simulink model "ur_servo"  (R2022b)
settings: Solver=FixedStepAuto  StartTime=0.0  StopTime=inf  RelTol=1e-3
model workspace (MAT data in the model file):
  SL_ROS_VariableLengthArrays_MaxSizes.CommonInfo.ArrayTruncateAction = 'EmitWarning'
  SL_ROS_VariableLengthArrays_MaxSizes.MsgTypeMap = containers.Map
  SL_ROS_VariableLengthArrays_MaxSizes.MsgTypeMap.serialization.keys = {'sensor_msgs/Image', 'std_msgs/Float64MultiArray', 'tf2_msgs/TFMessage'}
  SL_ROS_VariableLengthArrays_MaxSizes.MsgTypeMap.serialization.values{1}(1).PropertyName = 'Data'
  SL_ROS_VariableLengthArrays_MaxSizes.MsgTypeMap.serialization.values{1}(1).DataType = 'uint8'
  SL_ROS_VariableLengthArrays_MaxSizes.MsgTypeMap.serialization.values{1}(1).MaxLength = 921600
  SL_ROS_VariableLengthArrays_MaxSizes.MsgTypeMap.serialization.values{1}(2).PropertyName = 'Encoding'
  SL_ROS_VariableLengthArrays_MaxSizes.MsgTypeMap.serialization.values{1}(2).DataType = 'uint8'
  SL_ROS_VariableLengthArrays_MaxSizes.MsgTypeMap.serialization.values{1}(2).MaxLength = 921600
  SL_ROS_VariableLengthArrays_MaxSizes.MsgTypeMap.serialization.values{2}.PropertyName = 'Data'
  SL_ROS_VariableLengthArrays_MaxSizes.MsgTypeMap.serialization.values{2}.DataType = 'double'
  SL_ROS_VariableLengthArrays_MaxSizes.MsgTypeMap.serialization.values{2}.MaxLength = 16
  SL_ROS_VariableLengthArrays_MaxSizes.MsgTypeMap.serialization.values{3}.PropertyName = 'Transforms'
  SL_ROS_VariableLengthArrays_MaxSizes.MsgTypeMap.serialization.values{3}.DataType = 'geometry_msgs/TransformStamped'
  SL_ROS_VariableLengthArrays_MaxSizes.MsgTypeMap.serialization.values{3}.MaxLength = 1
  SL_ROS_VariableLengthArrays_MaxSizes.MsgTypeMap.serialization.uniformity = 0
  SL_ROS_VariableLengthArrays_MaxSizes.MsgTypeMap.serialization.keyType = 'char'
  SL_ROS_VariableLengthArrays_MaxSizes.MsgTypeMap.serialization.valueType = 'any'
undefined symbols (not defined in the file or in its folder): Angular, Linear
libraries: robotlib x10
settings Model: Creator=user  LastModifiedBy=16122
settings OptimizationCC: EnhancedBackFolding=on  PassReuseOutputArgsAs=Individual arguments  ZeroExternalMemoryAtStartup=off  ZeroInternalMemoryAtStartup=off  MaxStackSize=64  OptimizeBlockOrder=speed  DifferentSizesBufferReuse=on  OptimizationCustomize=off  EfficientTunableParamExpr=on
settings DebuggingCC: ParameterTunabilityLossMsg=error
settings HardwareCC: ProdBitPerPointer=32  ProdBitPerSizeT=32  ProdBitPerPtrDiffT=32  ProdLargestAtomicFloat=None  ProdIntDivRoundTo=Undefined  ProdEndianess=Unspecified  ProdWordSize=32  ProdHWDeviceType=Generic->Unspecified (assume 32-bit Generic)
settings SFSimCC: MATLABDynamicMemAlloc=off
settings RTWCC: Description=Embedded Coder  SystemTargetFile=ert.tlc  HardwareBoard=Robot Operating System (ROS)  TLCOptions="-aInlineSetEventsForThisBaseRateFcn=TLC_FALSE -aSuppressMultiTaskScheduler=TLC_FALSE  -aRateBasedStepFcn=0"  TemplateMakefile=ert_default_tmf  Toolchain=Catkin  TargetLang=C++
settings CodeAppCC: ForceParamTrailComments=on  IgnoreCustomStorageClasses=off  OperatorAnnotations=on  SimulinkDataObjDesc=on  SFDataObjDesc=on  InsertBlockDesc=on

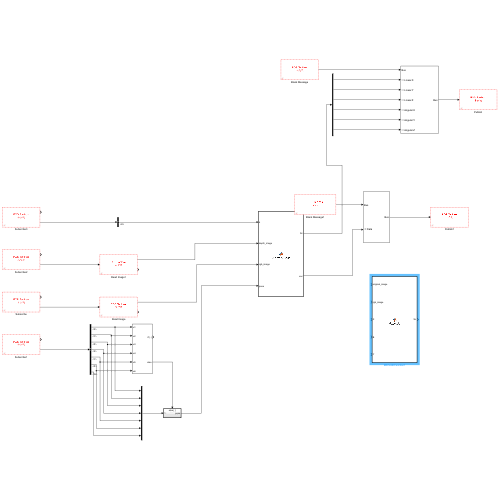
[thumbnail: Simulink's stored preview of the top-level diagram]
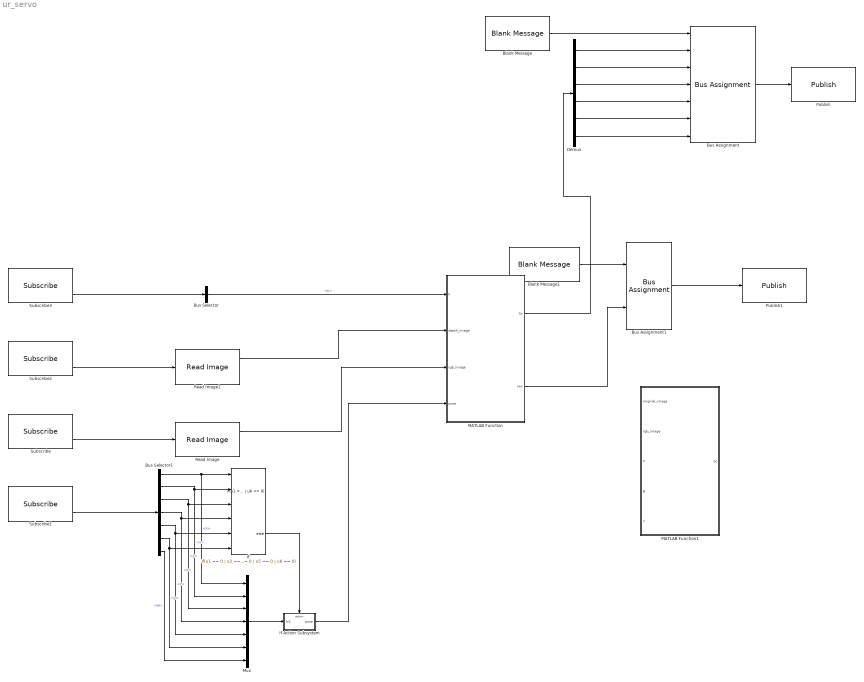
== system ur_servo ==
  Blank Message : robotlib/Blank Message  messageClass=Message  entityType=geometry_msgs/Twist  messageType=geometry_msgs/Twist  SampleTime=inf  legacyBusStruct=off
      settings: LibrarySourceBlock=roslib/ROS/Blank Message
  Blank Message1 : robotlib/Blank Message  messageClass=Message  entityType=std_msgs/Float64MultiArray  messageType=std_msgs/Float64MultiArray  SampleTime=inf  legacyBusStruct=off
      settings: LibrarySourceBlock=roslib/ROS/Blank Message
  Bus Assignment : BusAssignment  AssignedSignals=Linear.X,Linear.Y,Linear.Z,Angular.X,Angular.Y,Angular.Z
  Bus Assignment1 : BusAssignment  AssignedSignals=Data
  Bus Selector : BusSelector  OutputSignals=K
  Bus Selector1 : BusSelector  OutputSignals=Transforms.Transform.Translation.X,Transforms.Transform.Translation.Y,Transforms.Transform.Translation.Z,Transforms.Transform.Rotation.X,Transforms.Transform.Rotation.Y,Transforms.Transform.Rotation.Z,Transforms.Transform.Rotation.W
  Demux : Demux  Outputs=6
  If : If  NumInputs=6  IfExpression=u1 == 0 | u2 == 0 | u3 == 0 | u4 == 0 | u5 == 0 | u6 == 0
  If Action Subsystem : Subsystem  TreatAsAtomicUnit=on
  MATLAB Function : MATLAB Function  TreatAsAtomicUnit=on
  MATLAB Function1 : MATLAB Function  TreatAsAtomicUnit=on
  Mux : Mux  Inputs=7
  Publish : robotlib/Publish  topicSource=Select from ROS network  topic=/twist_controller/command  messageType=geometry_msgs/Twist  legacyBusStruct=off  messageQueueLength=1
      settings: LibrarySourceBlock=roslib/ROS/Publish
  Publish1 : robotlib/Publish  topicSource=Specify your own  topic=/urx  messageType=std_msgs/Float64MultiArray  legacyBusStruct=off  messageQueueLength=1
      settings: LibrarySourceBlock=roslib/ROS/Publish
  Read Image : robotlib/Read Image  MaximumImageSize=[480, 640]  ImageEncoding=rgb8  ShowAlphaOutput=off  ShowErrorCodeOutput=on  VariableSizeOutputs=off
      settings: LibrarySourceBlock=roslib/ROS/Read Image
  Read Image1 : robotlib/Read Image  MaximumImageSize=[480, 640]  ImageEncoding=16uc1  ShowAlphaOutput=off  ShowErrorCodeOutput=on  VariableSizeOutputs=off
      settings: LibrarySourceBlock=roslib/ROS/Read Image
  Subscribe : robotlib/Subscribe  topicSource=Select from ROS network  topic=/camera/color/image_raw  messageType=sensor_msgs/Image  SampleTime=-1  legacyBusStruct=off  messageQueueLength=1
      settings: LibrarySourceBlock=roslib/ROS/Subscribe
  Subscribe1 : robotlib/Subscribe  topicSource=Select from ROS network  topic=/tf  messageType=tf2_msgs/TFMessage  SampleTime=-1  legacyBusStruct=off  messageQueueLength=1
      settings: LibrarySourceBlock=roslib/ROS/Subscribe
  Subscribe2 : robotlib/Subscribe  topicSource=Select from ROS network  topic=/camera/aligned_depth_to_color/image_raw  messageType=sensor_msgs/Image  SampleTime=-1  legacyBusStruct=off  messageQueueLength=1
      settings: LibrarySourceBlock=roslib/ROS/Subscribe
  Subscribe3 : robotlib/Subscribe  topicSource=Select from ROS network  topic=/camera/color/camera_info  messageType=sensor_msgs/CameraInfo  SampleTime=-1  legacyBusStruct=off  messageQueueLength=1
      settings: LibrarySourceBlock=roslib/ROS/Subscribe
  wires:
  Subscribe/2 -> Read Image/1
  Read Image/1 -> MATLAB Function/3(rgb_image)
  Bus Selector1/1 -> Mux/1, If/1  "<X>"
  Bus Selector1/2 -> If/2, Mux/2  "<Y>"
  Bus Selector1/3 -> If/3, Mux/3  "<Z>"
  Bus Selector1/4 -> Mux/4, If/4  "<X>"
  Bus Selector1/5 -> Mux/5, If/5  "<Y>"
  Bus Selector1/6 -> If/6, Mux/6  "<Z>"
  If/2 -> If Action Subsystem/Action
  Subscribe2/2 -> Read Image1/1
  Read Image1/1 -> MATLAB Function/2(depth_image)
  Subscribe1/2 -> Bus Selector1/1
  Mux/1 -> If Action Subsystem/1(In1)
  If Action Subsystem/1(pose) -> MATLAB Function/4(pose)
  Subscribe3/2 -> Bus Selector/1
  Bus Selector/1 -> MATLAB Function/1(k)  "<K>"
  Blank Message/1 -> Bus Assignment/1
  Bus Assignment/1 -> Publish/1
  MATLAB Function/1(Sc) -> Demux/1
  Demux/1 -> Bus Assignment/2
  Demux/2 -> Bus Assignment/3
  Demux/3 -> Bus Assignment/4
  Demux/4 -> Bus Assignment/5
  Demux/5 -> Bus Assignment/6
  Demux/6 -> Bus Assignment/7
  Bus Selector1/7 -> Mux/7  "<W>"
  Blank Message1/1 -> Bus Assignment1/1
  MATLAB Function/2(vec) -> Bus Assignment1/2
  Bus Assignment1/1 -> Publish1/1

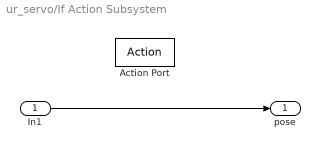
== system ur_servo/If Action Subsystem ==
  In1 : Inport
  Action Port : ActionPort  ActionPortLabel=else
  pose : Outport
  wires:
  In1/1 -> pose/1

== matlab function ur_servo/MATLAB Function1 ==
  data: original_image input; rgb_image input; Sc output; X input; B input; Y input
function Sc = call_get_I_z(original_image, rgb_image, X, B, Y)


% img = imread('img1.jpg');
% image_gray_old = rgb2gray(img);


% pose_T = [MatrixExp3(VecToso3(pose(4:6))), pose(1:3); 0 0 0 1];

% k = reshape(k, [3, 3]).';
image_gray_new = get_image_gray_norm(rgb2gray(rgb_image));
image_gray_old = get_image_gray_norm(rgb2gray(original_image));

[row, col] = size(rgb_image);
% [I_x, I_y] = get_image_gradient(image_gray, Para_Camera_Intrinsic);
% L_I = zeros(row*col, 6);
%% L_e
% cnt = 1;
for i = 1 : col
    for j = 1 : row
        

        point = [i; j; 1];
        corn_right_norm = Para_Camera_Intrinsic \ point;
        x = corn_right_norm(1);
        y = corn_right_norm(2);
%         Z_inv = planar_parameter' * corn_right_norm;
%         Z_inv = 1 / image_depth(j,i);
        L_I(cnt, :) = [I_x(j,i), ...
                       I_y(j,i), ...
                       I_z(j,i), ...
                       y * I_z(j,i), ...
                       -x * I_z(j,i), ...
                       x * I_y(j,i) - y * I_x(j,i)];
%         cnt = cnt + 1;
    end
end
% depth = double(depth_image) / 1000;
% [Sc, T] = servo_step_real(pose, image_gray_new, depth, k, image_gray_old);
% % vec = [T(1:3,4); AxisAng3(so3ToVec(MatrixLog3(T(1:3, 1:3))))]
% vec = reshape(T, [1, 16]);

end

== matlab function ur_servo/MATLAB Function ==
  data: k input; depth_image input; rgb_image input; pose input; Sc output; vec output
function [Sc, vec] = call_servo_step(k, depth_image, rgb_image, pose)

img = imread('img1.jpg');
image_gray_old = rgb2gray(img);


% pose_T = [MatrixExp3(VecToso3(pose(4:6))), pose(1:3); 0 0 0 1];

k = reshape(k, [3, 3]).';
image_gray_new = rgb2gray(rgb_image);
depth = double(depth_image) / 1000;
[Sc, T] = servo_step_real(pose, image_gray_new, depth, k, image_gray_old);
% vec = [T(1:3,4); AxisAng3(so3ToVec(MatrixLog3(T(1:3, 1:3))))]
vec = reshape(T, [1, 16]);

end
